simulink model "sample_level2_sfcn_block"  (Simulink 8.1)
settings: Solver=FixedStepDiscrete  StartTime=0.0  StopTime=inf  FixedStep=1/256  RelTol=1e-3
libraries: rt_clock_lib x1
settings Model: Creator=Irimia  LastModifiedBy=andre
settings DebuggingCC: FcnCallInpInsideContextMsg=EnableAllAsWarning
settings GRTTargetCC: CombineOutputUpdateFcns=on  GRTInterface=off

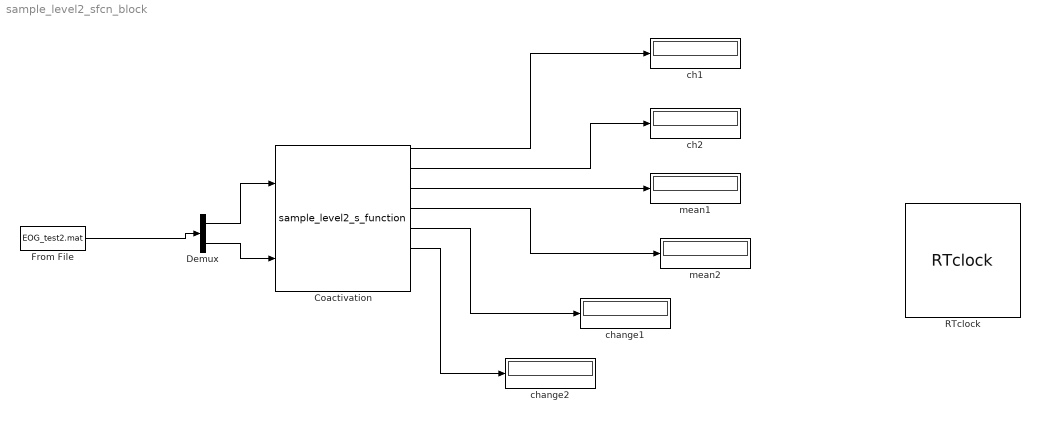
== system sample_level2_sfcn_block ==
  Coactivation : M-S-Function  FunctionName=sample_level2_s_function  Parameters=var1,var2  mask{var1=7, var2=0}
  Demux : Demux  Outputs=2
  From File : FromFile  FileName=EOG_test2.mat  SampleTime=1/256
  RTclock : rt_clock_lib/RTclock
  ch1 : Display
  ch2 : Display
  change1 : Display
  change2 : Display
  mean1 : Display
  mean2 : Display
  wires:
  Coactivation/1 -> ch1/1
  Coactivation/2 -> ch2/1
  Coactivation/3 -> mean1/1
  Coactivation/4 -> mean2/1
  Coactivation/5 -> change1/1
  Coactivation/6 -> change2/1
  From File/1 -> Demux/1
  Demux/2 -> Coactivation/2
  Demux/1 -> Coactivation/1
